simulink model "stein_hart"  (R2024a)
settings: Solver=FixedStepDiscrete  StartTime=0.0  StopTime=10  FixedStep=0.1  RelTol=1e-3
libraries: embreciprocals x2
settings Model: DataTypeOverride=Off  Creator=aptay  LastModifiedBy=aptay
settings SolverCC: AlgebraicLoopSolver=TrustRegion
settings DataIOCC: LimitDataPoints=on  SaveOutput=off  SaveTime=off
settings OptimizationCC: BlockReduction=off  ConditionallyExecuteInputs=off  DefaultParameterBehavior=Inlined  LifeSpan=inf
settings DebuggingCC: AlgebraicLoopMsg=error  SingleTaskRateTransMsg=error  UnconnectedInputMsg=warning  UnconnectedOutputMsg=warning  UnconnectedLineMsg=warning  AllowSymbolicDim=off  StrictBusMsg=ErrorOnBusTreatedAsVector  SFUnexpectedBacktrackingDiag=warning  SFNoUnconditionalDefaultTransitionDiag=warning  SFExecutionAtInitializationDiag=none  ArithmeticOperatorsInVariantConditions=warning
settings HardwareCC: ProdBitPerPointer=32  ProdBitPerSizeT=32  ProdBitPerPtrDiffT=32  ProdLargestAtomicFloat=None  ProdIntDivRoundTo=Undefined  ProdEndianess=Unspecified  ProdWordSize=32  ProdHWDeviceType=ASIC/FPGA->ASIC/FPGA  ProdEqTarget=off
settings ModelReferenceCC: EnableRefExpFcnMdlSchedulingChecks=on
settings SFSimCC: SimUseLocalCustomCode=off  CustomCodeUndefinedFunction=UseInterfaceOnly
settings RTWCC: RTWUseLocalCustomCode=off  GPUComputeCapability=3.5
settings CodeAppCC: StateflowObjectComments=on
settings GRTTargetCC: TargetLangStandard=C89/C90 (ANSI)
settings ConfigComp: CovScope=ReferencedModels  CovMetricSettings=dw  CovSaveCumulativeToWorkspaceVar=on  CovSaveSingleToWorkspaceVar=on  CovExternalEMLEnable=off  CovSFcnEnable=off

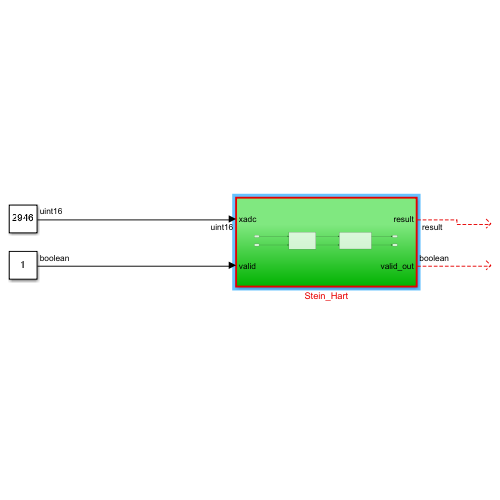
[thumbnail: Simulink's stored preview of the top-level diagram]
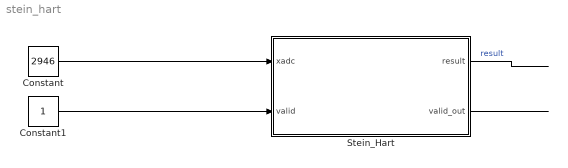
== system stein_hart ==
  Constant : Constant  Value=2946  OutMin=0  OutMax=4095  OutDataTypeStr=fixdt(0,16,0)  SampleTime=-1
  Constant1 : Constant  OutDataTypeStr=boolean  SampleTime=-1
  Stein_Hart : Subsystem  TreatAsAtomicUnit=on
  wires:
  Constant1/1 -> Stein_Hart/2(valid)
  Constant/1 -> Stein_Hart/1(xadc)
  Stein_Hart/1(result) -> ?  "result"
  Stein_Hart/2(valid_out) -> ?

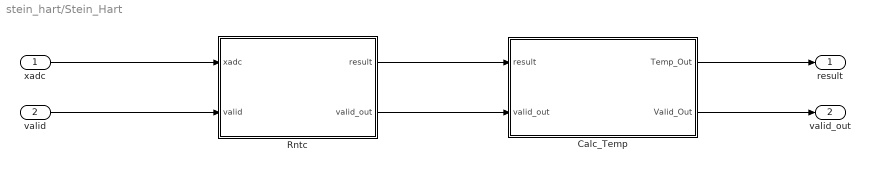
== system stein_hart/Stein_Hart ==
  xadc : Inport  OutMin=0  OutMax=4095  OutDataTypeStr=fixdt(0,16,0)
  valid : Inport  Port=2
  Calc_Temp : Subsystem
  Rntc : Subsystem
  result : Outport  VectorParamsAs1DForOutWhenUnconnected=off
  valid_out : Outport  Port=2  VectorParamsAs1DForOutWhenUnconnected=off
  wires:
  xadc/1 -> Rntc/1(xadc)
  valid/1 -> Rntc/2(valid)
  Calc_Temp/1(Temp_Out) -> result/1
  Calc_Temp/2(Valid_Out) -> valid_out/1
  Rntc/1(result) -> Calc_Temp/1(result)
  Rntc/2(valid_out) -> Calc_Temp/2(valid_out)

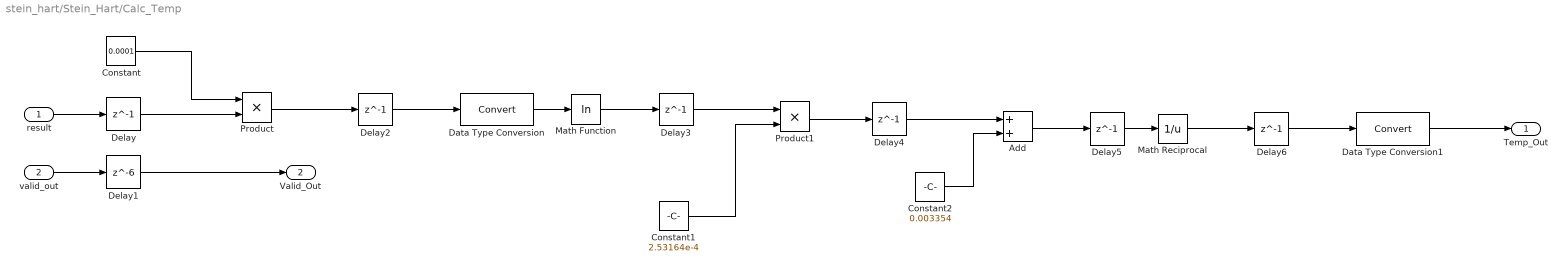
== system stein_hart/Stein_Hart/Calc_Temp ==
  result : Inport
  valid_out : Inport  Port=2
  Add : Sum
  Constant : Constant  Value=0.0001  OutMin=0.0001  OutMax=0.0001  OutDataTypeStr=fixdt(1,16,28)  SampleTime=-1
  Constant1 : Constant  Value=2.53164e-4  SampleTime=-1
  Constant2 : Constant  Value=0.003354  SampleTime=-1
  Data Type Conversion : DataTypeConversion  SaturateOnIntegerOverflow=off  RndMeth=Floor
  Data Type Conversion1 : DataTypeConversion  SaturateOnIntegerOverflow=off  RndMeth=Floor
  Delay{,2..6} (6 alike) : Delay  DelayLength=1  InitialCondition=0
  Delay1 : Delay  DelayLength=6  InitialCondition=0
  Math Function : Math  Operator=log  SignedPower=on  RndMeth=Zero
  Math Reciprocal : Math  Operator=reciprocal  SignedPower=on
  Product : Product
  Product1 : Product
  Temp_Out : Outport  OutDataTypeStr=fixdt(1,25,10)
  Valid_Out : Outport  Port=2  VectorParamsAs1DForOutWhenUnconnected=off
  wires:
  result/1 -> Delay/1
  valid_out/1 -> Delay1/1
  Delay/1 -> Product/2
  Constant/1 -> Product/1
  Product/1 -> Delay2/1
  Delay2/1 -> Data Type Conversion/1
  Data Type Conversion/1 -> Math Function/1
  Math Function/1 -> Delay3/1
  Constant1/1 -> Product1/2
  Product1/1 -> Delay4/1
  Constant2/1 -> Add/2
  Add/1 -> Delay5/1
  Math Reciprocal/1 -> Delay6/1
  Delay3/1 -> Product1/1
  Delay4/1 -> Add/1
  Delay5/1 -> Math Reciprocal/1
  Delay6/1 -> Data Type Conversion1/1
  Delay1/1 -> Valid_Out/1
  Data Type Conversion1/1 -> Temp_Out/1

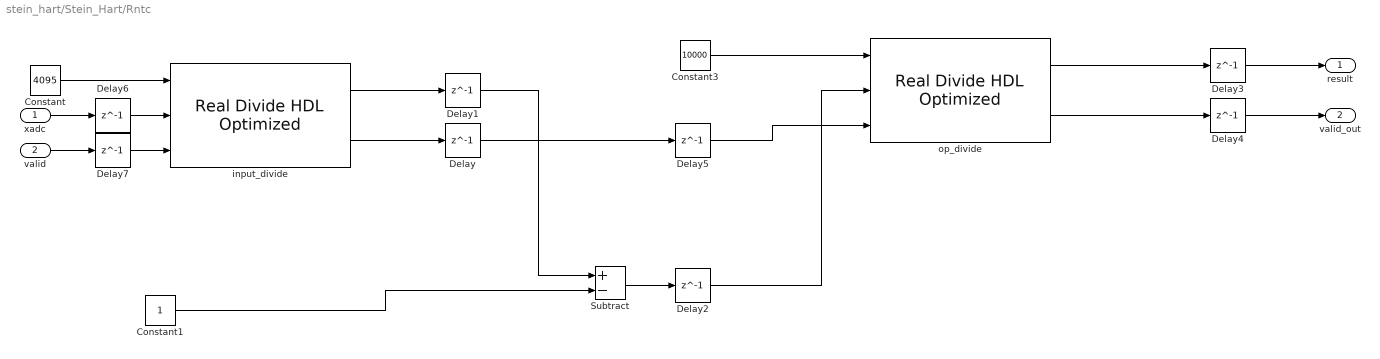
== system stein_hart/Stein_Hart/Rntc ==
  xadc : Inport  OutMin=0  OutMax=4095  OutDataTypeStr=fixdt(0,16,0)
  valid : Inport  Port=2
  Constant : Constant  Value=4095  OutDataTypeStr=fixdt(0,16,0)  SampleTime=-1
  Constant1 : Constant  OutDataTypeStr=fixdt(0,16,0)  SampleTime=-1
  Constant3 : Constant  Value=10000  OutMin=0  OutMax=10000  OutDataTypeStr=fixdt(1,25,10)  SampleTime=-1
  Delay{,1..7} (8 alike) : Delay  DelayLength=1  InitialCondition=0
  Subtract : Sum  Inputs=+-  OutDataTypeStr=fixdt(1,25,10, 'DataTypeOverride', 'Off')  AccumDataTypeStr=fixdt(1,18,10)
  input_divide : embreciprocals/Real Divide HDL Optimized  OutputType=fixdt(1,18,10)
      settings: LibrarySourceBlock=embeddedMatrixLib/Math Operations/Real Divide HDL Optimized
  op_divide : embreciprocals/Real Divide HDL Optimized  OutputType=fixdt(1,27,10)
      settings: LibrarySourceBlock=embeddedMatrixLib/Math Operations/Real Divide HDL Optimized
  result : Outport  VectorParamsAs1DForOutWhenUnconnected=off
  valid_out : Outport  Port=2  VectorParamsAs1DForOutWhenUnconnected=off
  wires:
  Constant/1 -> input_divide/1
  Constant3/1 -> op_divide/1
  op_divide/1 -> Delay3/1
  Constant1/1 -> Subtract/2
  op_divide/2 -> Delay4/1
  Delay7/1 -> input_divide/3
  xadc/1 -> Delay6/1
  Delay4/1 -> valid_out/1
  Delay2/1 -> op_divide/2
  Subtract/1 -> Delay2/1
  input_divide/1 -> Delay1/1
  valid/1 -> Delay7/1
  input_divide/2 -> Delay/1
  Delay3/1 -> result/1
  Delay1/1 -> Subtract/1
  Delay/1 -> Delay5/1
  Delay6/1 -> input_divide/2
  Delay5/1 -> op_divide/3
